simulink subsystem "Stanley_standfort_controller"  (R2022b)
settings: Solver=VariableStepAuto  StartTime=0.0  StopTime=10.0  RelTol=1e-3
undefined symbols (not defined in the file or in its folder): DiscIntNeverNeededParam
libraries: CarMaker4SL x4
settings Model: Creator=Admin  LastModifiedBy=Admin

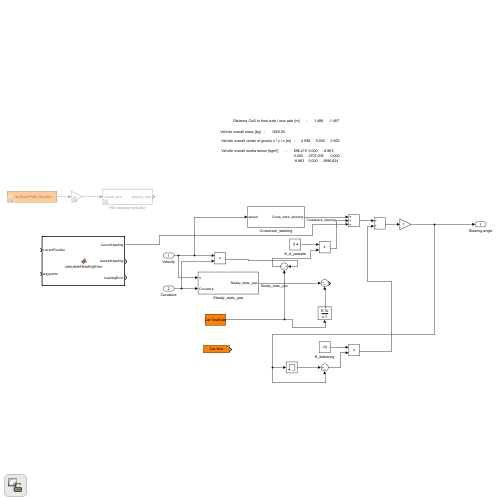
[thumbnail: Simulink's stored preview of the top-level diagram]
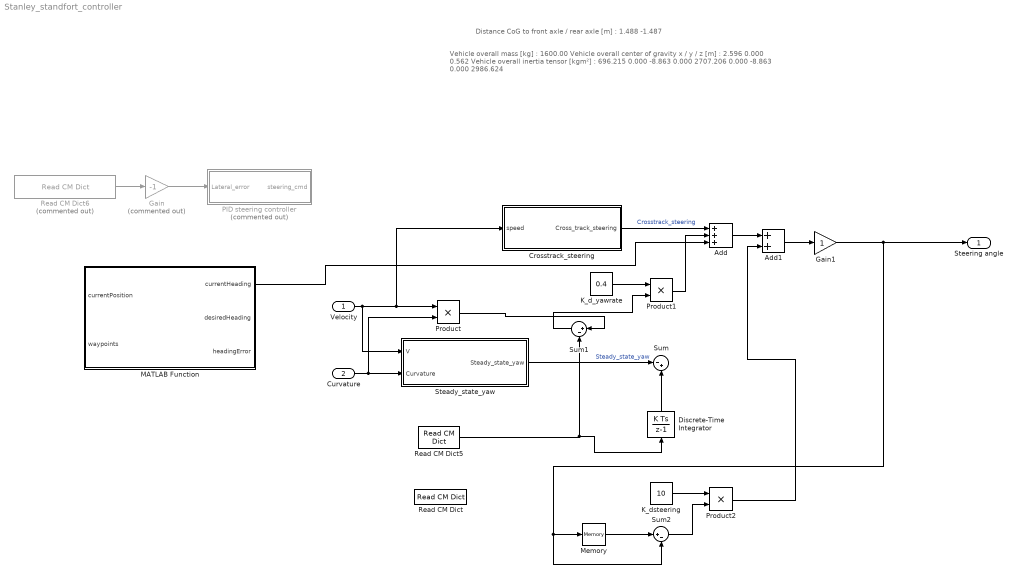
== system Stanley_standfort_controller ==
  note: Vehicle overall mass [kg] 	: 	1600.00
      |
      |  Vehicle overall center of gravity x / y / z [m] 	: 	2.596	0.000	0.562
      |
      |  Vehicle overall inertia tensor [kgm²] 	: 	696.215	0.000	-8.863
      |  	 									0.000	2707.206	0.000
      |  	 									-8.863	0.000	2986.624
  note: Distance CoG to front axle / rear axle [m] : 1.488 -1.487
  Velocity : Inport
  Curvature : Inport  Port=2
  Add : Sum  Inputs=+++
  Add1 : Sum
  Crosstrack_steering : Subsystem
  Discrete-Time Integrator : DiscreteIntegrator  SampleTime=-1  ICPrevOutput=DiscIntNeverNeededParam  ICPrevScaledInput=DiscIntNeverNeededParam
  Gain : Gain  Commented=on  Gain=-1
  Gain1 : Gain
  K_d_yawrate : Constant  Value=0.4
  K_dsteering : Constant  Value=10
  MATLAB Function : MATLAB Function  TreatAsAtomicUnit=on
  Memory : Memory  LinearizeAsDelay=on
  PID steering controller : Subsystem  Commented=on
  Product : Product
  Product1 : Product
  Product2 : Product
  Read CM Dict : CarMaker4SL/Read CM Dict  xname=Car.Yaw  xsync=off  xstime=Continuous
  Read CM Dict5 : CarMaker4SL/Read CM Dict  xname=Car.YawRate  xsync=off  xstime=Continuous
  Read CM Dict6 : CarMaker4SL/Read CM Dict  Commented=on  xname=Car.Road.Path.DevDist  xsync=off  xstime=Continuous
  Steady_state_yaw : Subsystem
  Sum : Sum  Inputs=|-+
  Sum1 : Sum  Inputs=|+-
  Sum2 : Sum  Inputs=|+-
  Steering angle : Outport
  wires:
  Steady_state_yaw/1(Steady_state_yaw) -> Sum/1  "Steady_state_yaw"
  Product/1 -> Sum1/1
  Read CM Dict6/1 -> Gain/1
  Velocity/1 -> Steady_state_yaw/1(V), Crosstrack_steering/1(speed), Product/1
  Curvature/1 -> Product/2, Steady_state_yaw/2(Curvature)
  Gain/1 -> PID steering controller/1(Lateral_error)
  Read CM Dict5/1 -> Discrete-Time Integrator/1, Sum1/2
  Crosstrack_steering/1(Cross_track_steering) -> Add/1  "Crosstrack_steering"
  Sum1/1 -> Product1/2
  K_d_yawrate/1 -> Product1/1
  Memory/1 -> Sum2/1
  Product1/1 -> Add/2
  Add/1 -> Add1/1
  K_dsteering/1 -> Product2/1
  Sum2/1 -> Product2/2
  Add1/1 -> Gain1/1
  Product2/1 -> Add1/2
  Gain1/1 -> Steering angle/1, Memory/1, Sum2/2
  MATLAB Function/1(currentHeading) -> Add/3
  Discrete-Time Integrator/1 -> Sum/2

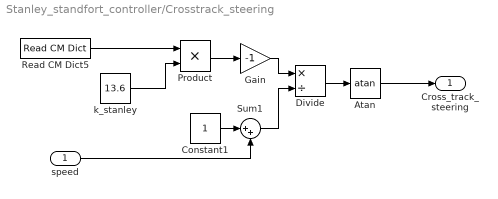
== system Stanley_standfort_controller/Crosstrack_steering ==
  speed : Inport
  Atan : Trigonometry  Operator=atan
  Constant1 : Constant
  Divide : Product  Inputs=*/
  Gain : Gain  Gain=-1
  Product : Product
  Read CM Dict5 : CarMaker4SL/Read CM Dict  xname=Car.Road.Path.DevDist  xsync=off  xstime=Continuous
  Sum1 : Sum  Inputs=|++
  k_stanley : Constant  Value=13.6
  Cross_track_steering : Outport
  wires:
  Gain/1 -> Divide/1
  Read CM Dict5/1 -> Product/1
  Product/1 -> Gain/1
  Sum1/1 -> Divide/2
  k_stanley/1 -> Product/2
  speed/1 -> Sum1/2
  Constant1/1 -> Sum1/1
  Divide/1 -> Atan/1
  Atan/1 -> Cross_track_steering/1

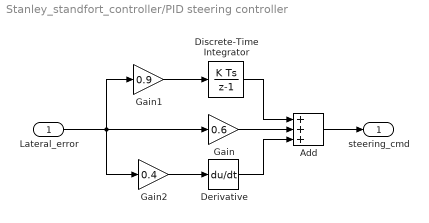
== system Stanley_standfort_controller/PID steering controller ==
  Lateral_error : Inport
  Add : Sum  Inputs=+++
  Derivative : Derivative
  Discrete-Time Integrator : DiscreteIntegrator  SampleTime=-1  ICPrevOutput=DiscIntNeverNeededParam  ICPrevScaledInput=DiscIntNeverNeededParam
  Gain : Gain  Gain=0.6
  Gain1 : Gain  Gain=0.9
  Gain2 : Gain  Gain=0.4
  steering_cmd : Outport
  wires:
  Add/1 -> steering_cmd/1
  Derivative/1 -> Add/3
  Gain/1 -> Add/2
  Gain1/1 -> Discrete-Time Integrator/1
  Gain2/1 -> Derivative/1
  Discrete-Time Integrator/1 -> Add/1
  Lateral_error/1 -> Gain2/1, Gain/1, Gain1/1

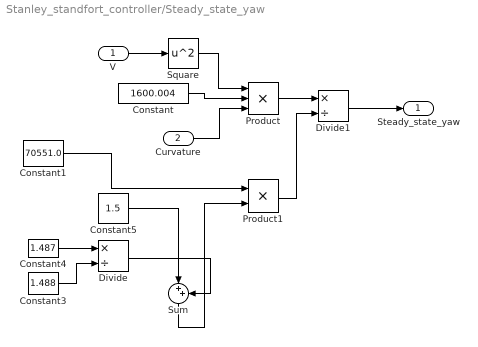
== system Stanley_standfort_controller/Steady_state_yaw ==
  V : Inport
  Curvature : Inport  Port=2
  Constant : Constant  Value=1600.004
  Constant1 : Constant  Value=70551.0
  Constant3 : Constant  Value=1.488
  Constant4 : Constant  Value=1.487
  Constant5 : Constant  Value=1.5
  Divide : Product  Inputs=*/
  Divide1 : Product  Inputs=*/
  Product : Product  Inputs=3
  Product1 : Product
  Square : Math  Operator=square
  Sum : Sum  Inputs=|++
  Steady_state_yaw : Outport
  wires:
  Divide1/1 -> Steady_state_yaw/1
  Product1/1 -> Divide1/2
  Product/1 -> Divide1/1
  Constant1/1 -> Product1/1
  Curvature/1 -> Product/3
  Constant/1 -> Product/2
  Sum/1 -> Product1/2
  Divide/1 -> Sum/2
  V/1 -> Square/1
  Constant3/1 -> Divide/2
  Constant5/1 -> Sum/1
  Constant4/1 -> Divide/1
  Square/1 -> Product/1

== matlab function Stanley_standfort_controller/MATLAB Function ==
  data: currentPosition input; currentHeading output; waypoints input; desiredHeading output; headingError output
function [currentHeading, desiredHeading, headingError] = calculateHeadingError(currentPosition, waypoints)
    % Calculate current heading, desired heading, and heading error for Stanley controller
    % Inputs:
    %   - currentPosition: Current position of the vehicle [x, y] (in a 2D plane)
    %   - waypoints: Array of waypoints [x, y] representing the desired path
    % Outputs:
    %   - currentHeading: Current heading of the vehicle (in radians)
    %   - desiredHeading: Desired heading or reference angle (in radians)
    %   - headingError: Heading error (in radians)
    
    function angle = wrapToPi(angle)
    % Wrap angle to the range [-pi, pi]
    angle = mod(angle + pi, 2 * pi) - pi;
    end

    % Extract x and y coordinates from the current position
    x = currentPosition(1);
    y = currentPosition(2);

    % Find the nearest waypoint on the path
    [~, index] = min(sum((waypoints - [x, y]).^2, 2));
    nearestWaypoint = waypoints(index, :);

    % Calculate the vector from the vehicle to the nearest waypoint
    headingVector = nearestWaypoint - [x, y];

    % Calculate the current heading
    currentHeading = atan2(headingVector(2), headingVector(1));

    % Calculate the desired heading (heading of the vector between the current and next waypoints)
    if index < size(waypoints, 1)
        nextWaypoint = waypoints(index + 1, :);
    else
        % If the vehicle is at the last waypoint, use the previous waypoint as the next waypoint
        nextWaypoint = waypoints(end - 1, :);
    end
    desiredHeading = atan2(nextWaypoint(2) - nearestWaypoint(2), nextWaypoint(1) - nearestWaypoint(1));

    % Calculate heading error
    headingError = wrapToPi(desiredHeading - currentHeading);
end
